simulink model "motor_characterization"  (R2016b)
settings: Solver=VariableStepAuto  StartTime=0.0  StopTime=10.0  RelTol=1e-3
model workspace (MAT data in the model file):
  thrust_table = Simulink.LookupTable
  thrust_table.Table = Simulink.lookuptable.Table
  thrust_table.Table.Value = [0.106891 0.110024 0.113157 0.11629 0.119423 0.122556 0.125689 0.128822 0.131955 0.135088 0.138221 0.141354 ... (734 elements, 1x734)]
  thrust_table.Table.Dimensions = [1 734]
  thrust_table.Table.DataType = 'auto'
  thrust_table.Table.FieldName = 'Table'
  thrust_table.Breakpoints = Simulink.lookuptable.Breakpoint
  thrust_table.Breakpoints.Value = [1127 1128 1129 1130 1131 1132 1133 1134 1135 1136 1137 1138 ... (734 elements, 1x734)]
  thrust_table.Breakpoints.TunableSizeName = 'N1'
  thrust_table.Breakpoints.Dimensions = [1 734]
  thrust_table.Breakpoints.DataType = 'auto'
  thrust_table.Breakpoints.FieldName = 'BP1'
  thrust_table.SupportTunableSize = 0
  thrust_table.StructTypeInfo = Simulink.lookuptable.StructTypeInfo
  thrust_table.StructTypeInfo.Name = 'thrust_table_st_def'
  thrust_table.StructTypeInfo.DataScope = 'Auto'
settings Model: Creator=Dylan  LastModifiedBy=Dylan

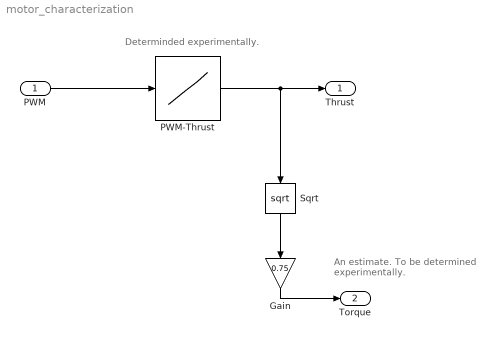
== system motor_characterization ==
  note: An estimate.  To be determined
      | experimentally.
  note: Determinded experimentally.
  "PWM " : Inport
  Gain : Gain  Gain=0.75
  "PWM-Thrust " : Lookup_n-D  NumberOfTableDimensions=1  DataSpecification=Lookup table object  LookupTableObject=thrust_table  BreakpointsForDimension1=[-5:5]  Table=tanh([-5:5])  InternalRulePriority=Speed  RndMeth=Simplest  InputSameDT=on
  Sqrt : Sqrt  SaturateOnIntegerOverflow=on
  "Thrust " : Outport
  Torque : Outport  Port=2
  wires:
  "PWM "/1 -> "PWM-Thrust "/1
  "PWM-Thrust "/1 -> Sqrt/1, "Thrust "/1
  Sqrt/1 -> Gain/1
  Gain/1 -> Torque/1
